simulink library "xrbsControl_r3"  (Simulink 5.0)
undefined symbols (not defined in the file or in its folder): xlDistRamDepth, xlMatrixToOutputVec, xlMatrixToStateInitVec, xlNumMealyElements, xlNumMooreOutputElements, xlNumMooreStateElements, xlNumStateBits, xlRegMealyInitVec
libraries: xbsIndex_r3 x13
settings Model: Creator=singhj  LastModifiedBy=singhj

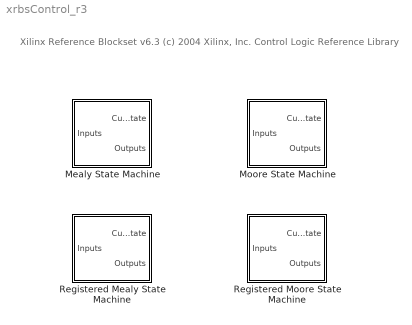
== system xrbsControl_r3 ==
  note: Xilinx Reference Blockset v6.3
      | (c) 2004  Xilinx, Inc.
      |
      | Control Logic Reference Library
  Mealy State Machine : Subsystem  mask(Xilinx Mealy State Machine){next_state_matrix=[0 1; 2 1; 0 3; 2 1], output_matrix=[0 0; 0 0; 0 0; 0 1], n_bits=1, period=1}
      mask prompts: next_state_matrix "Next State Matrix"; output_matrix "Output Matrix"; n_bits "Number of  Output Bits"; period "Sample Period"
      mask help: Implements a Mealy state machine. The output is a function of the current state and input.
      mask init:
      | % Set Block Logo
      | [bg,fg] = xlcmap('XBlock',0);
      | iPos = get_param(gcb,'Position');
      | iWidth=iPos(3)-iPos(1); iHeight=iPos(4)-iPos(2);
      | iCx=iWidth/2;
      | iCy=iHeight/2;
      | [logoX, logoY] = xlogo(iPos);
      mask Help: web(xlhtmldoclink('Mealy State Machine'));
      mask Display:
      | patch([0 iWidth iWidth 0],[0 0 iHeight iHeight] , bg);
      | patch(logoX,logoY, fg);
      | port_label('input',1,'Inputs');
      | port_label('output',1,'CurrentState');
      | port_label('output',2,'Outputs');
      | 
      | plot([0 0 iWidth iWidth 0], [0 iHeight iHeight 0 0]);
  Moore State Machine : Subsystem  mask(Xilinx Moore State Machine){next_state_matrix=[0 1; 2 1; 0 3; 2 4; 0 1], output_matrix=[0; 0; 0; 0; 1], n_bits=1, period=1}
      mask prompts: next_state_matrix "Next State Matrix"; output_matrix "Output Array"; n_bits "Number of Output Bits"; period "Sample Period"
      mask help: Implements a Moore state machine. The output is a function only of the current state.
      mask init:
      | % Set Block Logo
      | [bg,fg] = xlcmap('XBlock',0);
      | iPos = get_param(gcb,'Position');
      | iWidth=iPos(3)-iPos(1); iHeight=iPos(4)-iPos(2);
      | iCx=iWidth/2;
      | iCy=iHeight/2;
      | [logoX, logoY] = xlogo(iPos);
      mask Help: web(xlhtmldoclink('Moore State Machine'));
      mask Display:
      | patch([0 iWidth iWidth 0],[0 0 iHeight iHeight] , bg);
      | patch(logoX,logoY, fg);
      | port_label('input',1,'Inputs');
      | port_label('output',1,'CurrentState');
      | port_label('output',2,'Outputs');
      | 
      | plot([0 0 iWidth iWidth 0], [0 iHeight iHeight 0 0]);
  Registered Mealy State Machine : Subsystem  mask(Xilinx Registered Mealy State Machine){next_state_matrix=[0 1; 2 1; 0 3; 2 1], output_matrix=[0 0; 0 0; 0 0; 0 1], n_bits=1, period=1}
      mask prompts: next_state_matrix "Next State Matrix"; output_matrix "Output Matrix"; n_bits "Number of Output Bits"; period "Sample Period"
      mask help: Implements a registered Mealy state machine. The output is a function of the current state and its input. The output is registered.
      mask init:
      | % Set Block Logo
      | [bg,fg] = xlcmap('XBlock',0);
      | iPos = get_param(gcb,'Position');
      | iWidth=iPos(3)-iPos(1); iHeight=iPos(4)-iPos(2);
      | iCx=iWidth/2;
      | iCy=iHeight/2;
      | [logoX, logoY] = xlogo(iPos);
      mask Help: web(xlhtmldoclink('Registered Mealy State Machine'));
      mask Display:
      | patch([0 iWidth iWidth 0],[0 0 iHeight iHeight] , bg);
      | patch(logoX,logoY, fg);
      | port_label('input',1,'Inputs');
      | port_label('output',1,'CurrentState');
      | port_label('output',2,'Outputs');
      | 
      | plot([0 0 iWidth iWidth 0], [0 iHeight iHeight 0 0]);
  Registered Moore State Machine : Subsystem  mask(Xilinx Registered Moore State Machine){next_state_matrix=[0 1; 2 1; 0 3; 2 4; 0 1], output_matrix=[0; 0; 0; 0; 1], n_bits=1, period=1}
      mask prompts: next_state_matrix "Next State Matrix"; output_matrix "Output Array"; n_bits "Number of Output Bits"; period "Sample Period"
      mask help: Implements a registered Moore state machine. The output is a function only of the current state. The output is registered.
      mask init:
      | % Set Block Logo
      | [bg,fg] = xlcmap('XBlock',0);
      | iPos = get_param(gcb,'Position');
      | iWidth=iPos(3)-iPos(1); iHeight=iPos(4)-iPos(2);
      | iCx=iWidth/2;
      | iCy=iHeight/2;
      | [logoX, logoY] = xlogo(iPos);
      mask Help: web(xlhtmldoclink('Registered Moore State Machine'));
      mask Display:
      | patch([0 iWidth iWidth 0],[0 0 iHeight iHeight] , bg);
      | patch(logoX,logoY, fg);
      | port_label('input',1,'Inputs');
      | port_label('output',1,'CurrentState');
      | port_label('output',2,'Outputs');
      | 
      | plot([0 0 iWidth iWidth 0], [0 iHeight iHeight 0 0]);

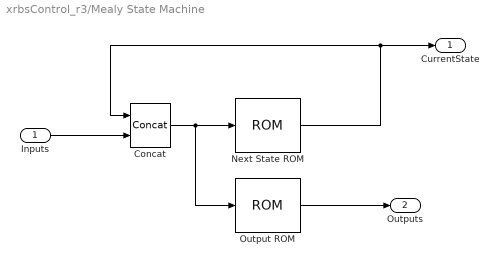
== system xrbsControl_r3/Mealy State Machine ==
  Inputs : Inport
  Concat : xbsIndex_r3/Concat  explicit_period=off  period=1  dbl_ovrd=off
  Next State ROM : xbsIndex_r3/ROM  depth=xlNumMealyElements(next_state_matrix, output_matrix)  initVector=xlMatrixToStateInitVec(next_state_matrix,xlNumStateBits(next_state_matrix),0,1,1,1)  arith_type=Unsigned  n_bits=xlNumStateBits(next_state_matrix)  bin_pt=0  latency=1  distributed_mem=off  init_zero=on  explicit_period=on  period=period  en=off  dbl_ovrd=off  gen_core=on  use_rpm=off
      settings: xl_area=[0, 0, 0, 0, 0, 0, 0]
  Output ROM : xbsIndex_r3/ROM  depth=xlDistRamDepth(output_matrix)  initVector=xlMatrixToOutputVec(output_matrix,n_bits,0,1,1,1)  arith_type=Unsigned  n_bits=n_bits  bin_pt=0  latency=0  distributed_mem=on  init_zero=on  explicit_period=on  period=period  en=off  dbl_ovrd=off  gen_core=on  use_rpm=off
      settings: xl_area=[0, 0, 0, 0, 0, 0, 0]
  CurrentState : Outport
  Outputs : Outport  Port=2
  wires:
  Inputs/1 -> Concat/2
  Output ROM/1 -> Outputs/1
  Concat/1 -> Next State ROM/1, Output ROM/1
  Next State ROM/1 -> Concat/1, CurrentState/1

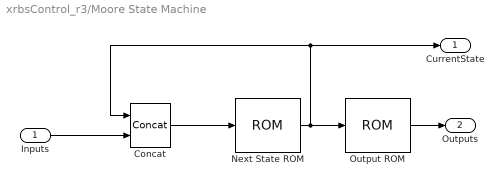
== system xrbsControl_r3/Moore State Machine ==
  Inputs : Inport
  Concat : xbsIndex_r3/Concat  explicit_period=off  period=1  dbl_ovrd=off
  Next State ROM : xbsIndex_r3/ROM  depth=xlNumMooreStateElements(next_state_matrix, output_matrix)  initVector=xlMatrixToStateInitVec(next_state_matrix,xlNumStateBits(next_state_matrix),0,1,1,1)  arith_type=Unsigned  n_bits=xlNumStateBits(next_state_matrix)  bin_pt=0  latency=1  distributed_mem=off  init_zero=on  explicit_period=on  period=period  en=off  dbl_ovrd=off  gen_core=on  use_rpm=off
      settings: xl_area=[0, 0, 0, 0, 0, 0, 0]
  Output ROM : xbsIndex_r3/ROM  depth=xlDistRamDepth(output_matrix)  initVector=xlMatrixToOutputVec(output_matrix,n_bits,0,1,1,1)  arith_type=Unsigned  n_bits=n_bits  bin_pt=0  latency=0  distributed_mem=on  init_zero=on  explicit_period=on  period=period  en=off  dbl_ovrd=off  gen_core=on  use_rpm=off
      settings: xl_area=[0, 0, 0, 0, 0, 0, 0]
  CurrentState : Outport
  Outputs : Outport  Port=2
  wires:
  Inputs/1 -> Concat/2
  Output ROM/1 -> Outputs/1
  Concat/1 -> Next State ROM/1
  Next State ROM/1 -> Concat/1, CurrentState/1, Output ROM/1

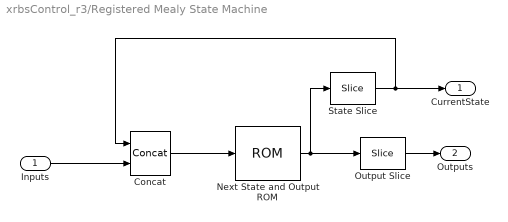
== system xrbsControl_r3/Registered Mealy State Machine ==
  Inputs : Inport
  Concat : xbsIndex_r3/Concat  explicit_period=off  period=1  dbl_ovrd=off
  Next State and Output ROM : xbsIndex_r3/ROM  depth=xlNumMealyElements(next_state_matrix, output_matrix)  initVector=xlRegMealyInitVec(next_state_matrix, output_matrix, n_bits,0,1,1,1)  arith_type=Unsigned  n_bits=xlNumStateBits(next_state_matrix)+n_bits  bin_pt=0  latency=1  distributed_mem=off  init_zero=on  explicit_period=on  period=period  en=off  dbl_ovrd=off  gen_core=on  use_rpm=off
      settings: xl_area=[0, 0, 0, 0, 0, 0, 0]
  Output Slice : xbsIndex_r3/Slice  mode=Lower Bit Location + Width  nbits=n_bits  bit1=0  base1=MSB of Input  bit0=0  base0=LSB of Input  boolean_output=off  explicit_period=off  period=1  dbl_ovrd=off
  State Slice : xbsIndex_r3/Slice  mode=Upper Bit Location + Width  nbits=xlNumStateBits(next_state_matrix)  bit1=0  base1=MSB of Input  bit0=0  base0=LSB of Input  boolean_output=off  explicit_period=off  period=1  dbl_ovrd=off
  CurrentState : Outport
  Outputs : Outport  Port=2
  wires:
  Inputs/1 -> Concat/2
  Output Slice/1 -> Outputs/1
  Concat/1 -> Next State and Output ROM/1
  Next State and Output ROM/1 -> Output Slice/1, State Slice/1
  State Slice/1 -> CurrentState/1, Concat/1

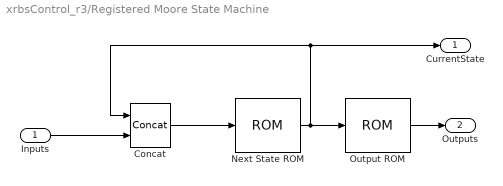
== system xrbsControl_r3/Registered Moore State Machine ==
  Inputs : Inport
  Concat : xbsIndex_r3/Concat  explicit_period=off  period=1  dbl_ovrd=off
  Next State ROM : xbsIndex_r3/ROM  depth=xlNumMooreStateElements(next_state_matrix, output_matrix)  initVector=xlMatrixToStateInitVec(next_state_matrix,xlNumStateBits(next_state_matrix),0,1,1,1)  arith_type=Unsigned  n_bits=xlNumStateBits(next_state_matrix)  bin_pt=0  latency=1  distributed_mem=off  init_zero=on  explicit_period=on  period=period  en=off  dbl_ovrd=off  gen_core=on  use_rpm=off
      settings: xl_area=[0, 0, 0, 0, 0, 0, 0]
  Output ROM : xbsIndex_r3/ROM  depth=xlNumMooreOutputElements(output_matrix)  initVector=xlMatrixToOutputVec(output_matrix,n_bits,0,1,1,1)  arith_type=Unsigned  n_bits=n_bits  bin_pt=0  latency=1  distributed_mem=off  init_zero=on  explicit_period=on  period=period  en=off  dbl_ovrd=off  gen_core=on  use_rpm=off
      settings: xl_area=[0, 0, 0, 0, 0, 0, 0]
  CurrentState : Outport
  Outputs : Outport  Port=2
  wires:
  Next State ROM/1 -> Output ROM/1, CurrentState/1, Concat/1
  Concat/1 -> Next State ROM/1
  Output ROM/1 -> Outputs/1
  Inputs/1 -> Concat/2
